simulink model "qbmove_example"  (R2019a)
settings: Solver=ode1  StartTime=0.0  StopTime=inf  FixedStep=.0005  RelTol=1e-3  EnableMultiTasking=on
libraries: qbmove_library x2, simulink x2, QB_pacer_lib x1
settings Model: Creator=laurentio  LastModifiedBy=alextoind
settings DataIOCC: LimitDataPoints=on  SaveFormat=Array  ReturnWorkspaceOutputs=off
settings OptimizationCC: LifeSpan=inf
settings DebuggingCC: UnderspecifiedInitializationDetection=Classic  MergeDetectMultiDrivingBlocksExec=none  SolverPrmCheckMsg=warning  AllowSymbolicDim=off  StateNameClashWarn=warning  SFUnexpectedBacktrackingDiag=warning  SFNoUnconditionalDefaultTransitionDiag=warning  SFExecutionAtInitializationDiag=none  ArithmeticOperatorsInVariantConditions=warning
settings HardwareCC: ProdBitPerPointer=32  ProdBitPerSizeT=32  ProdBitPerPtrDiffT=32  ProdLargestAtomicFloat=None  ProdIntDivRoundTo=Undefined  ProdEndianess=Unspecified  ProdWordSize=32  ProdHWDeviceType=32-bit Generic
settings ModelReferenceCC: PropagateSignalLabelsOutOfModel=off
settings SFSimCC: SimUseLocalCustomCode=off
settings RTWCC: RTWUseLocalCustomCode=off
settings CodeAppCC: StateflowObjectComments=on
settings GRTTargetCC: TargetLangStandard=C89/C90 (ANSI)  GeneratePreprocessorConditionals=Disable all
settings ConfigComp: CovMetricSettings=dw  CovHtmlReporting=on  CovSaveCumulativeToWorkspaceVar=on  CovSaveSingleToWorkspaceVar=on  CovExternalEMLEnable=off  CovSFcnEnable=off

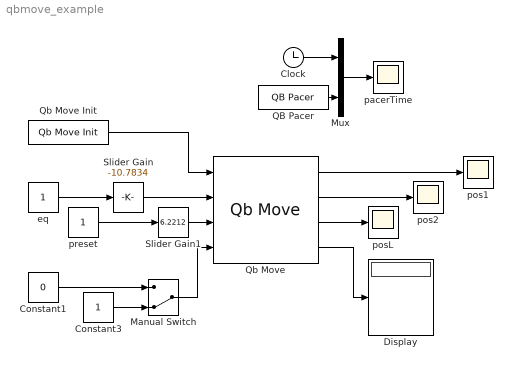
== system qbmove_example ==
  Clock : Clock
  Constant1 : Constant  Value=0
  Constant3 : Constant
  Display : Display
  Manual Switch : ManualSwitch  CurrentSetting=0
  Mux : Mux  Inputs=2
  QB Pacer : QB_pacer_lib/QB Pacer  simTimePerRealTime=1
  Qb Move : qbmove_library/Qb Move  ID=[3]  ACTIVE_COMM_DIRECTIONS=Both  CONTROL_MODE=Equilibrium Position and Stiffness Preset  DAISY_CHAINING=off  MAX_ANG=0  SW_LIMIT=inf  OFFSET=0  ACTIVATE=off  WDT=0.0  UNIT=Degrees
      settings: SourceProductName=Qb Move Library
  Qb Move Init : qbmove_library/Qb Move Init  NUMBER_OF_COM='/dev/ttyUSB0'  BAUD_RATE_COM=2000000
      settings: SourceProductName=Qb Move Library
  Slider Gain : simulink/Math Operations/Slider Gain  gain=-10.7834  low=-180  high=180
  "Slider Gain1 " : simulink/Math Operations/Slider Gain  gain=6.2212  low=0  high=30
  eq : Constant
  pacerTime : Scope
  pos1 : Scope
  pos2 : Scope
  posL : Scope
  preset : Constant
  wires:
  QB Pacer/1 -> Mux/2
  Clock/1 -> Mux/1
  Qb Move Init/1 -> Qb Move/1
  eq/1 -> Slider Gain/1
  preset/1 -> "Slider Gain1 "/1
  Constant1/1 -> Manual Switch/1
  Slider Gain/1 -> Qb Move/2
  Constant3/1 -> Manual Switch/2
  "Slider Gain1 "/1 -> Qb Move/3
  Qb Move/4 -> Display/1
  Mux/1 -> pacerTime/1
  Manual Switch/1 -> Qb Move/4
  Qb Move/1 -> pos1/1
  Qb Move/2 -> pos2/1
  Qb Move/3 -> posL/1
